simulink library "Prop_demo"  (R2025b)
settings: Solver=VariableStepAuto  StartTime=0.0  StopTime=10.0  RelTol=1e-3
undefined symbols (not defined in the file): cfd2d_ja, cfd2d_jl, cfd2d_kQ, cfd2d_kT, cfd2d_P1_CEF_X, cfd2d_P1_CEF_Y, cfd2d_P1_CEF_Z, cfd2d_P1_CEM_X, cfd2d_P1_CEM_Y, cfd2d_P1_CEM_Z, cfd3d_ja, cfd3d_jl, cfd3d_P2_CEF_X, cfd3d_P2_CEF_Y, cfd3d_P2_CEF_Z, cfd3d_P2_CEM_X, cfd3d_P2_CEM_Y, cfd3d_P2_CEM_Z, cfd3d_pitch, CoefBus, DF3000_V2_Prop, magnitude, Prop1, Prop2
libraries: simulink_extras x7, matrix_library x3, sharedtransform x3, simulink x2, DF3000_V2_Common x1
(part 1 of 2)
settings Model: Creator=someone  LastModifiedBy=someone

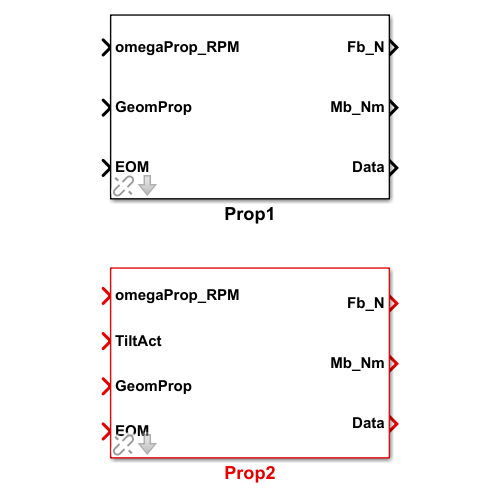
[thumbnail: Simulink's stored preview of the top-level diagram]
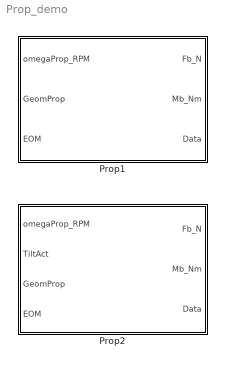
== system Prop_demo ==
  Prop1 : Subsystem  AncestorBlock=DF3000_V2_Prop/Prop1  mask{propAbs=1}
      mask prompts: propAbs "Prop Index"
      mask DialogControl ParameterGroupVar Prompt: 参数
  Prop2 : Subsystem  AncestorBlock=DF3000_V2_Prop/Prop2  mask{propAbs=2, ArmDirSelected=on}
      mask prompts: propAbs "Prop Index"; ArmDirSelected "Positive Installed (Front Prop)"
      mask DialogControl ParameterGroupVar Prompt: 参数

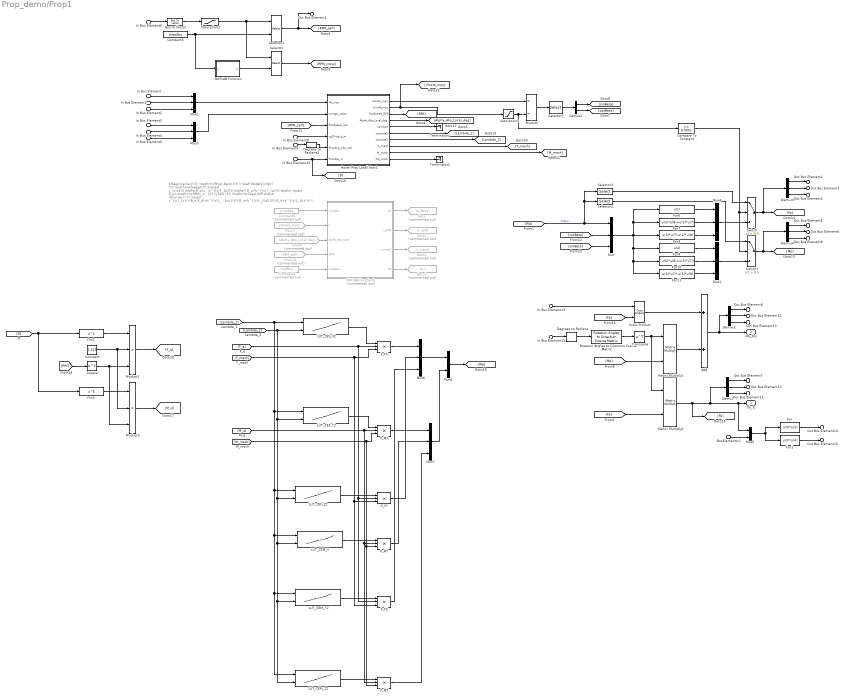
== system Prop_demo/Prop1 ==
  note: $\begin{array}{l} \mathrm{Prop\ Aero\ Fit\ /\ Coef\ Model}\\[3pt] (1)\ \mathrm{Sweep\ fit:}\quad y_{c,p}(V,\alpha,R_p)=a^{(c)}_{p}(V,\alpha)\,R_p+b^{(c)}_{p}(V,\alpha),\quad R_p=\mathrm{RPM}_p^{2}.\\[5pt] (2)\ \mathrm{Coax\ diff\ plane\ (one\ pair):}\\ \quad y^{u}_{c}(V,R_u,R_d)=k^{(c)}_{uu}(V)\,R_u+k^{(c)}_{ud}(V)\,R_d+b^{(c)}_{u}(V),\\ \quad y^{d}_{c}(V,R_u,R_d)=k^{(c)}_{du}(V)\,R_u+k^{(c)}_{dd}(V)\,R_d+b^{(c)}_{d}(V).\\[5pt] (3)\ \mathrm{Ratio\ (split\ of\ slope):}\quad s^{(c)}_{u}=k^{(c)}_{uu}+k^{(c)}_{ud},\quad s^{(c)}_{d}=k^{(c)}_{dd}+k^{(c)}_{du},\\ \quad r^{(c)}_{uu}=\frac{k^{(c)}_{uu}}{s^{(c)}_{u}},\quad r^{(c)}_{ud}=\frac{k^{(c)}_{ud}}{s^{(c)}_{u}},\quad r^{(c)}_{dd}=\frac{k^{(c)}_{dd}}{s^{(c)}_{d}},\quad r^{(c)}_{du}=\frac{k^{(c)}_{du}}{s^{(c)}_{d}}.\\[5pt] (4)\ \mathrm{Coax\ weight:}\quad s=(\cos(\alpha))^{p},\quad p=\mathrm{coaxAlphaPow}.\\ \quad \mathrm{upper:}\quad a^{(c)}_{\mathrm{self}}=s\,r^{(c)}_{uu}\,a^{(c)}_{p},\quad a^{(c)}_{\mathrm{cross}}=s\,r^{(c)}_{ud}\,a^{(c)}_{p},\\ \quad \mathrm{lower:}\quad a^{(c)}_{\mathrm{self}}=s\,r^{(c)}_{dd}\,a^{(c)}_{p},\quad a^{(c)}_{\mathrm{cross}}=s\,r^{(c)}_{du}\,a^{(c)}_{p}.\\[5pt] (5)\ \mathrm{Final\ prediction:}\quad \hat y_{c,p}=a^{(c)}_{\mathrm{self}}\,R_p+a^{(c)}_{\mathrm{cross}}\,R_{m(p)}+b^{(c)}_{p}(V,\alpha). \end{array}$
  In Bus Element6 : Inport  PortName=omegaProp_RPM
      settings: AttributesFormatString=%<OutDataTypeStr>\nDimensions: %<PortDimensions>
  In Bus Element12 : Inport  Port=2  PortName=GeomProp  Element=cg2Prop_b_m
      settings: AttributesFormatString=%<OutDataTypeStr>\nDimensions: %<PortDimensions>
  In Bus Element8 : Inport  Port=2  PortName=GeomProp  Element=cg2Prop_b_m
      settings: AttributesFormatString=%<OutDataTypeStr>\nDimensions: %<PortDimensions>
  In Bus Element13 : Inport  Port=2  PortName=GeomProp  Element=PropAng_b2p_deg
      settings: AttributesFormatString=%<OutDataTypeStr>\nDimensions: %<PortDimensions>
  In Bus Element9 : Inport  Port=2  PortName=GeomProp  Element=PropAng_b2p_deg
      settings: AttributesFormatString=%<OutDataTypeStr>\nDimensions: %<PortDimensions>
  In Bus Element10 : Inport  Port=2  PortName=GeomProp  Element=PropDia_m
      settings: AttributesFormatString=%<OutDataTypeStr>\nDimensions: %<PortDimensions>
  BusElementIn1 : Inport  Port=2  PortName=GeomProp  Element=root2Prop_b_m
  In Bus Element : Inport  Port=3  PortName=EOM  Element=VB_mps.Ub_mps
      settings: AttributesFormatString=%<OutDataTypeStr>\nDimensions: %<PortDimensions>
  In Bus Element1 : Inport  Port=3  PortName=EOM  Element=VB_mps.Vb_mps
      settings: AttributesFormatString=%<OutDataTypeStr>\nDimensions: %<PortDimensions>
  In Bus Element2 : Inport  Port=3  PortName=EOM  Element=VB_mps.Wb_mps
      settings: AttributesFormatString=%<OutDataTypeStr>\nDimensions: %<PortDimensions>
  In Bus Element3 : Inport  Port=3  PortName=EOM  Element=Rates_radps.P_radps
      settings: AttributesFormatString=%<OutDataTypeStr>\nDimensions: %<PortDimensions>
  In Bus Element4 : Inport  Port=3  PortName=EOM  Element=Rates_radps.Q_radps
      settings: AttributesFormatString=%<OutDataTypeStr>\nDimensions: %<PortDimensions>
  In Bus Element5 : Inport  Port=3  PortName=EOM  Element=Rates_radps.R_radps
      settings: AttributesFormatString=%<OutDataTypeStr>\nDimensions: %<PortDimensions>
  Add : Sum
  Bus to Vector : BusToVector
  Compare To Constant : simulink/Logic and Bit Operations/Compare To Constant  relop=<=  const=0.0001  OutDataTypeStr=boolean
  Constant : Constant  Value=1.225
  Constant3 : Constant  Value=propAbs
  Constant4 : Constant  Commented=on  Value=CoefBus  OutDataTypeStr=Bus: CoefBusObj
  Constant5 : Constant  Commented=on  Value=propAbs
  Cross Product : matrix_library/Cross Product
  Degrees to Radians : simulink_extras/Transformations/Degrees to Radians
  Degrees to Radians1 : simulink_extras/Transformations/Degrees to Radians
  Demux{,2..4} (4 alike) : Demux  Outputs=3
  Demux1 : Demux  Outputs=2
  Fcn : Fcn  Expr=u(3)*u(5)
  Fcn1 : Fcn  Expr=u(3)*u(4)
  Fcn10 : Fcn  Expr=u(6)*u(8)+u(5)*u(7)
  Fcn11 : Fcn  Expr=u(6)*u(7)-u(5)*u(8)
  Fcn2 : Fcn  Expr=u^4
  Fcn3 : Fcn  Expr=u^5
  Fcn6 : Fcn  Expr=u(1)
  Fcn7 : Fcn  Expr=u(3)*u(8)+u(2)*u(7)
  Fcn8 : Fcn  Expr=u(3)*u(7)-u(2)*u(8)
  Fcn9 : Fcn  Expr=u(4)
  From14 : From  Commented=on  GotoTag=RPM_self
  From6 : From  Commented=on  GotoTag=Alpha_Abs_Local_deg
  From7 : From  Commented=on  GotoTag=Vmold_mps
  Goto : Goto  Commented=on  GotoTag=a_base
  Goto1 : Goto  Commented=on  GotoTag=r_self
  Goto2 : Goto  Commented=on  GotoTag=r_cross
  Goto3 : Goto  Commented=on  GotoTag=b
  Hover Prop Local Vars1 : Subsystem  AncestorBlock=DF3000_V2_Common/Hover Prop Local Vars1
  LUT_CEF_X2 : Lookup_n-D  BreakpointsForDimension1=cfd2d_ja  BreakpointsForDimension2=cfd2d_jl  BreakpointsForDimension3=[5, 7]  Table=cfd2d_P1_CEF_X  ExtrapMethod=Clip  UseLastTableValue=on  InternalRulePriority=Speed  RndMeth=Simplest
      settings: InputPortMap=u0,u1
  LUT_CEF_Y2 : Lookup_n-D  BreakpointsForDimension1=cfd2d_ja  BreakpointsForDimension2=cfd2d_jl  BreakpointsForDimension3=[5, 7]  Table=cfd2d_P1_CEM_X  ExtrapMethod=Clip  UseLastTableValue=on  InternalRulePriority=Speed  RndMeth=Simplest
      settings: InputPortMap=u0,u1
  LUT_CEF_Z2 : Lookup_n-D  BreakpointsForDimension1=cfd2d_ja  BreakpointsForDimension2=cfd2d_jl  BreakpointsForDimension3=[5, 7]  Table=cfd2d_P1_CEF_Y  ExtrapMethod=Clip  UseLastTableValue=on  InternalRulePriority=Speed  RndMeth=Simplest
      settings: InputPortMap=u0,u1
  LUT_CEM_X : Lookup_n-D  BreakpointsForDimension1=cfd2d_ja  BreakpointsForDimension2=cfd2d_jl  BreakpointsForDimension3=[5, 7]  Table=cfd2d_P1_CEM_Y  ExtrapMethod=Clip  UseLastTableValue=on  InternalRulePriority=Speed  RndMeth=Simplest
      settings: InputPortMap=u0,u1
  LUT_CEM_Y2 : Lookup_n-D  BreakpointsForDimension1=cfd2d_ja  BreakpointsForDimension2=cfd2d_jl  BreakpointsForDimension3=[5, 7]  Table=cfd2d_P1_CEF_Z  ExtrapMethod=Clip  UseLastTableValue=on  InternalRulePriority=Speed  RndMeth=Simplest
      settings: InputPortMap=u0,u1
  LUT_CEM_Z2 : Lookup_n-D  BreakpointsForDimension1=cfd2d_ja  BreakpointsForDimension2=cfd2d_jl  BreakpointsForDimension3=[5, 7]  Table=cfd2d_P1_CEM_Z  ExtrapMethod=Clip  UseLastTableValue=on  InternalRulePriority=Speed  RndMeth=Simplest
      settings: InputPortMap=u0,u1
  MATLAB Function : MATLAB Function  TreatAsAtomicUnit=on
  MATLAB Function2 : MATLAB Function  Commented=on  TreatAsAtomicUnit=on
  Matrix Multiply1 : Product  Multiplication=Matrix(*)
  Matrix Multiply2 : Product  Multiplication=Matrix(*)
  Mux{,1..4,6..7} (7 alike) : Mux  Inputs=3
  Mux5 : Mux  Inputs=2
  Mux8 : Mux  Inputs=2
  P_FX : Product  Inputs=***
  P_FY : Product  Inputs=***
  P_FZ : Product  Inputs=***
  P_MX : Product  Inputs=***
  P_MY : Product  Inputs=***
  P_MZ : Product  Inputs=***
  Product : Product  Inputs=*/
  Product1 : Product  Inputs=3
  Product3 : Product  Inputs=3
  Rotation Angles to Direction Cosine Matrix : sharedtransform/Rotation Angles to Direction Cosine Matrix  rotationOrder=XYZ  aMode=aMode
  Saturation1 : Saturate  UpperLimit=inf  LowerLimit=0.0001
  Saturation2 : Saturate  UpperLimit=1500  LowerLimit=0
      settings: AttributesFormatString=min: %<LowerLimit>\nmax: %<UpperLimit>
  Selector : Selector  InputPortWidth=8  IndexOptions=Index vector (port)  Indices=[1 3]  OutputSizes=1
  Selector1 : Selector  InputPortWidth=8  IndexOptions=Index vector (port)  Indices=[1 3]  OutputSizes=1
  Selector2 : Selector  InputPortWidth=3  IndexOptions=Index vector (dialog)  Indices=[2 3]  OutputSizes=1
  Selector3 : Selector  InputPortWidth=6  IndexOptions=Index vector (dialog)  Indices=[1 2 3]  OutputSizes=1
  Selector4 : Selector  InputPortWidth=6  IndexOptions=Index vector (dialog)  Indices=[4 5 6]  OutputSizes=1
  Square : Math  Operator=square
  Switch : Switch  Criteria=u2 > Threshold  Threshold=0.5  SaturateOnIntegerOverflow=off  InputSameDT=off
  Switch1 : Switch  Criteria=u2 > Threshold  Threshold=0.5  SaturateOnIntegerOverflow=off  InputSameDT=off
  Terminator1 : Terminator
  Terminator2 : Terminator
  Transpose : Math  Operator=transpose
  Fb_N : Outport  PortDimensions=3
  Mb_Nm : Outport  Port=2  PortDimensions=3
  Out Bus Element7 : Outport  Port=3  PortName=Data  Element=Fx_Prop
  Out Bus Element10 : Outport  Port=3  PortName=Data  Element=Fy_Prop
  Out Bus Element11 : Outport  Port=3  PortName=Data  Element=Fz_Prop
  Out Bus Element8 : Outport  Port=3  PortName=Data  Element=Mx_Prop
  Out Bus Element12 : Outport  Port=3  PortName=Data  Element=My_Prop
  Out Bus Element13 : Outport  Port=3  PortName=Data  Element=Mz_Prop
  Out Bus Element1 : Outport  Port=3  PortName=Data  Element=RPM
  Out Bus Element2 : Outport  Port=3  PortName=Data  Element=Fx_Local
  Out Bus Element3 : Outport  Port=3  PortName=Data  Element=Fy_Local
  Out Bus Element4 : Outport  Port=3  PortName=Data  Element=Fz_Local
  Out Bus Element5 : Outport  Port=3  PortName=Data  Element=Mx_Local
  Out Bus Element6 : Outport  Port=3  PortName=Data  Element=My_Local
  Out Bus Element9 : Outport  Port=3  PortName=Data  Element=Mz_Local
  Out Bus Element14 : Outport  Port=3  PortName=Data  Element=BMbx_Prop
  Out Bus Element15 : Outport  Port=3  PortName=Data  Element=BMby_Prop
  wires:
  Fcn1/1 -> Out Bus Element15/1
  Fcn/1 -> Out Bus Element14/1
  Mux5/1 -> Fcn/1, Fcn1/1
  BusElementIn1/1 -> Mux5/2
  From14/1 -> MATLAB Function2/4(RPM)
  Demux4/2 -> Out Bus Element6/1
  Demux4/1 -> Out Bus Element5/1
  Demux4/3 -> Out Bus Element9/1
  Demux3/3 -> Out Bus Element4/1
  Demux3/1 -> Out Bus Element2/1
  Demux3/2 -> Out Bus Element3/1
  Selector3/1 -> Switch/1
  Switch/1 -> [Fp], Demux3/1
  Selector4/1 -> Switch1/1
  Mux4/1 -> Switch/3
  Saturation1/1 -> Product/2, Compare To Constant/1
  Compare To Constant/1 -> Switch/2, Switch1/2
  Mux1/1 -> Switch1/3
  Switch1/1 -> [Mp], Demux4/1
  Demux1/1 -> [sinBeta]
  Demux1/2 -> [cosBeta]
  Selector/1 -> [RPM_cross]
  MATLAB Function/1(y) -> Selector/2
  Constant3/1 -> Selector1/2, MATLAB Function/1(u)
  In Bus Element6/1 -> Bus to Vector/1
  Bus to Vector/1 -> Saturation2/1
  Saturation2/1 -> Selector/1, Selector1/1
  MATLAB Function2/1(a6) -> Goto/1
  Rotation Angles to Direction Cosine Matrix/1 -> Transpose/1
  In Bus Element12/1 -> Cross Product/1
  Cross Product/1 -> Add/1
  In Bus Element13/1 -> Degrees to Radians/1
  Degrees to Radians/1 -> Rotation Angles to Direction Cosine Matrix/1
  Matrix Multiply1/1 -> Add/2
  [Mp] -> Matrix Multiply1/2
  Transpose/1 -> Matrix Multiply2/1, Matrix Multiply1/1
  Selector1/1 -> [RPM_self], Out Bus Element1/1
  In Bus Element8/1 -> Hover Prop Local Vars1/4(cg2Prop_b_m)
  In Bus Element9/1 -> Degrees to Radians1/1
  In Bus Element/1 -> Mux2/1
  In Bus Element5/1 -> Mux3/3
  In Bus Element4/1 -> Mux3/2
  In Bus Element3/1 -> Mux3/1
  In Bus Element2/1 -> Mux2/3
  In Bus Element10/1 -> [D], Hover Prop Local Vars1/6(PropDia_m)
  Mux3/1 -> Hover Prop Local Vars1/2(omega_radps)
  Mux2/1 -> Hover Prop Local Vars1/1(Vb_mps)
  In Bus Element1/1 -> Mux2/2
  [RPM_self] -> Hover Prop Local Vars1/3(RotSpeed_rpm)
  Hover Prop Local Vars1/1(VLocal_mps) -> Product/1
  Hover Prop Local Vars1/2(Vmold_mps) -> [Vmold_mps], Saturation1/1
  Product/1 -> Selector2/1
  Selector2/1 -> Demux1/1
  Hover Prop Local Vars1/3(RotSpeed_RPS) -> [RPS]
  Hover Prop Local Vars1/5(Lambda) -> Terminator1/1
  Constant4/1 -> MATLAB Function2/5(CoefBus)
  Constant5/1 -> MATLAB Function2/1(propAbs)
  MATLAB Function2/4(b6) -> Goto3/1
  MATLAB Function2/3(r_cross6) -> Goto2/1
  MATLAB Function2/2(r_self6) -> Goto1/1
  Hover Prop Local Vars1/4(Alpha_Abs_Local_deg) -> [Alpha_Abs_Local_deg]
  From6/1 -> MATLAB Function2/3(Alpha_abs_local)
  From7/1 -> MATLAB Function2/2(V)
  [cosBeta] -> Mux/2
  [sinBeta] -> Mux/3
  Mux/1 -> Fcn7/1, Fcn6/1, Fcn10/1, Fcn11/1, Fcn9/1, Fcn8/1
  Fcn9/1 -> Mux1/1
  Fcn10/1 -> Mux1/2
  Fcn11/1 -> Mux1/3
  Fcn6/1 -> Mux4/1
  Fcn7/1 -> Mux4/2
  Fcn8/1 -> Mux4/3
  [Fp] -> Matrix Multiply2/2
  Matrix Multiply2/1 -> Demux/1, Fb_N/1, Mux5/1, [Fb]
  [Fb] -> Cross Product/2
  [Wp] -> Mux/1, Selector3/1, Selector4/1  "FMpw"
  Demux/1 -> Out Bus Element7/1
  Demux/2 -> Out Bus Element10/1
  Demux/3 -> Out Bus Element11/1
  Demux2/3 -> Out Bus Element13/1
  Demux2/2 -> Out Bus Element12/1
  Demux2/1 -> Out Bus Element8/1
  Add/1 -> Mb_Nm/1, Demux2/1
  Degrees to Radians1/1 -> Hover Prop Local Vars1/5(PropAng_b2p_rad)
  [RPS] -> Square/1
  Square/1 -> Product3/3, Product1/3
  Product3/1 -> [M_q]
  Constant/1 -> Product3/2, Product1/2
  Product1/1 -> [F_q]
  Fcn2/1 -> Product1/1
  Fcn3/1 -> Product3/1
  LUT_CEM_Z2/1 -> P_MZ/1
  LUT_CEF_Z2/1 -> P_FY/1
  [M_q] -> P_MZ/2, P_MY/2, P_MX/2
  [M_mach] -> P_MZ/3, P_MY/3, P_MX/3
  LUT_CEF_X2/1 -> P_FX/1
  LUT_CEM_Y2/1 -> P_FZ/1
  [Lambda_1] -> LUT_CEM_Z2/1, LUT_CEM_Y2/1, LUT_CEM_X/1, LUT_CEF_Z2/1, LUT_CEF_Y2/1, LUT_CEF_X2/1
  P_FX/1 -> Mux6/1
  [Lambda_2] -> LUT_CEM_Z2/2, LUT_CEM_Y2/2, LUT_CEM_X/2, LUT_CEF_Z2/2, LUT_CEF_Y2/2, LUT_CEF_X2/2
  LUT_CEM_X/1 -> P_MY/1
  P_MX/1 -> Mux7/1
  LUT_CEF_Y2/1 -> P_MX/1
  [F_mach] -> P_FZ/3, P_FY/3, P_FX/3
  [F_q] -> P_FZ/2, P_FY/2, P_FX/2
  Hover Prop Local Vars1/6(Lambda1) -> [Lambda_1]
  Hover Prop Local Vars1/7(Lambda2) -> [Lambda_2]
  Hover Prop Local Vars1/8(F_mach) -> [F_mach]
  Hover Prop Local Vars1/9(M_mach) -> [M_mach]
  Hover Prop Local Vars1/10(Tip_mach) -> Terminator2/1
  P_FY/1 -> Mux6/2
  P_FZ/1 -> Mux6/3
  P_MY/1 -> Mux7/2
  P_MZ/1 -> Mux7/3
  Mux6/1 -> Mux8/1
  Mux7/1 -> Mux8/2
  Mux8/1 -> [Wp]
  [D] -> Fcn3/1, Fcn2/1

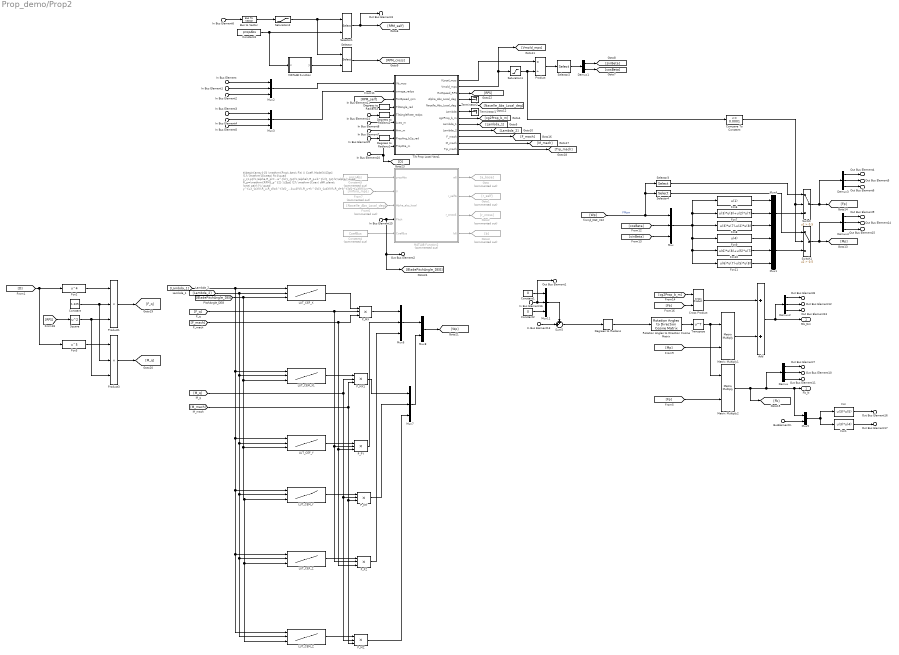
== system Prop_demo/Prop2 ==
  note: $\begin{array}{l} \mathrm{Prop\ Aero\ Fit\ /\ Coef\ Model}\\[3pt] (1)\ \mathrm{Sweep\ fit:}\quad y_{c,p}(V,\alpha,R_p)=a^{(c)}_{p}(V,\alpha)\,R_p+b^{(c)}_{p}(V,\alpha),\quad R_p=\mathrm{RPM}_p^{2}.\\[5pt] (2)\ \mathrm{Coax\ diff\ plane\ (one\ pair):}\\ \quad y^{u}_{c}(V,R_u,R_d)=k^{(c)}_{uu}(V)\,R_u+k^{(c)}_{ud}(V)\,R_d+b^{(c)}_{u}(V),\\ \quad y^{d}_{c}(V,R_u,R_d)=k^{(c)}_{du}(V)\,R_u+k^{(c)}_{dd}(V)\,R_d+b^{(c)}_{d}(V).\\[5pt] (3)\ \mathrm{Ratio\ (split\ of\ slope):}\quad s^{(c)}_{u}=k^{(c)}_{uu}+k^{(c)}_{ud},\quad s^{(c)}_{d}=k^{(c)}_{dd}+k^{(c)}_{du},\\ \quad r^{(c)}_{uu}=\frac{k^{(c)}_{uu}}{s^{(c)}_{u}},\quad r^{(c)}_{ud}=\frac{k^{(c)}_{ud}}{s^{(c)}_{u}},\quad r^{(c)}_{dd}=\frac{k^{(c)}_{dd}}{s^{(c)}_{d}},\quad r^{(c)}_{du}=\frac{k^{(c)}_{du}}{s^{(c)}_{d}}.\\[5pt] (4)\ \mathrm{Coax\ weight:}\quad s=(\cos(\alpha))^{p},\quad p=\mathrm{coaxAlphaPow}.\\ \quad \mathrm{upper:}\quad a^{(c)}_{\mathrm{self}}=s\,r^{(c)}_{uu}\,a^{(c)}_{p},\quad a^{(c)}_{\mathrm{cross}}=s\,r^{(c)}_{ud}\,a^{(c)}_{p},\\ \quad \mathrm{lower:}\quad a^{(c)}_{\mathrm{self}}=s\,r^{(c)}_{dd}\,a^{(c)}_{p},\quad a^{(c)}_{\mathrm{cross}}=s\,r^{(c)}_{du}\,a^{(c)}_{p}.\\[5pt] (5)\ \mathrm{Final\ prediction:}\quad \hat y_{c,p}=a^{(c)}_{\mathrm{self}}\,R_p+a^{(c)}_{\mathrm{cross}}\,R_{m(p)}+b^{(c)}_{p}(V,\alpha). \end{array}$
  In Bus Element6 : Inport  PortName=omegaProp_RPM
      settings: AttributesFormatString=%<OutDataTypeStr>\nDimensions: %<PortDimensions>
  In Bus Element14 : Inport  Port=2  PortName=TiltAct  Element=TiltAngleRate_dps
  In Bus Element15 : Inport  Port=2  PortName=TiltAct  Element=BladePitchAngle_DEG
  In Bus Element11 : Inport  Port=2  PortName=TiltAct  Element=TiltAngle_DEG
  In Bus Element16 : Inport  Port=2  PortName=TiltAct  Element=TiltAngle_DEG
  In Bus Element13 : Inport  Port=3  PortName=GeomProp  Element=PropAng_b2p_deg
      settings: AttributesFormatString=%<OutDataTypeStr>\nDimensions: %<PortDimensions>
  In Bus Element9 : Inport  Port=3  PortName=GeomProp  Element=PropAng_b2p_deg
      settings: AttributesFormatString=%<OutDataTypeStr>\nDimensions: %<PortDimensions>
  In Bus Element10 : Inport  Port=3  PortName=GeomProp  Element=PropDia_m
      settings: AttributesFormatString=%<OutDataTypeStr>\nDimensions: %<PortDimensions>
  In Bus Element8 : Inport  Port=3  PortName=GeomProp  Element=cg2PropHinge_b_m
      settings: AttributesFormatString=%<OutDataTypeStr>\nDimensions: %<PortDimensions>
  BusElementIn : Inport  Port=3  PortName=GeomProp  Element=cg2PropHinge_b_m
  In Bus Element7 : Inport  Port=3  PortName=GeomProp  Element=TiltArm_m
      settings: AttributesFormatString=%<OutDataTypeStr>\nDimensions: %<PortDimensions>
  In Bus Element : Inport  Port=4  PortName=EOM  Element=VB_mps.Ub_mps
      settings: AttributesFormatString=%<OutDataTypeStr>\nDimensions: %<PortDimensions>
  In Bus Element1 : Inport  Port=4  PortName=EOM  Element=VB_mps.Vb_mps
      settings: AttributesFormatString=%<OutDataTypeStr>\nDimensions: %<PortDimensions>
  In Bus Element2 : Inport  Port=4  PortName=EOM  Element=VB_mps.Wb_mps
      settings: AttributesFormatString=%<OutDataTypeStr>\nDimensions: %<PortDimensions>
  In Bus Element3 : Inport  Port=4  PortName=EOM  Element=Rates_radps.P_radps
      settings: AttributesFormatString=%<OutDataTypeStr>\nDimensions: %<PortDimensions>
  In Bus Element4 : Inport  Port=4  PortName=EOM  Element=Rates_radps.Q_radps
      settings: AttributesFormatString=%<OutDataTypeStr>\nDimensions: %<PortDimensions>
  In Bus Element5 : Inport  Port=4  PortName=EOM  Element=Rates_radps.R_radps
      settings: AttributesFormatString=%<OutDataTypeStr>\nDimensions: %<PortDimensions>
  Add : Sum
  Bus to Vector : BusToVector
  Compare To Constant : simulink/Logic and Bit Operations/Compare To Constant  relop=<=  const=0.0001  OutDataTypeStr=boolean
  Constant : Constant  Value=1.225
  Constant1 : Constant  Value=0
  Constant2 : Constant  Value=0
  Constant3 : Constant  Value=propAbs
  Constant4 : Constant  Commented=on  Value=CoefBus  OutDataTypeStr=Bus: CoefBusObj
  Constant5 : Constant  Commented=on  Value=propAbs
  Cross Product : matrix_library/Cross Product
  Degrees to Radians{,1..3} (4 alike) : simulink_extras/Transformations/Degrees to Radians
  Demux{,2..4} (4 alike) : Demux  Outputs=3
  Demux1 : Demux  Outputs=2
  Fcn : Fcn  Expr=u(3)*u(5)
  Fcn1 : Fcn  Expr=u(3)*u(4)
  Fcn10 : Fcn  Expr=u(6)*u(8)+u(5)*u(7)
  Fcn11 : Fcn  Expr=u(6)*u(7)-u(5)*u(8)
  Fcn2 : Fcn  Expr=u^4
  Fcn3 : Fcn  Expr=u^5
  Fcn6 : Fcn  Expr=u(1)
  Fcn7 : Fcn  Expr=u(3)*u(8)+u(2)*u(7)
  Fcn8 : Fcn  Expr=u(3)*u(7)-u(2)*u(8)
  Fcn9 : Fcn  Expr=u(4)
  From6 : From  Commented=on  GotoTag=Nacelle_Abs_Local_deg
  From7 : From  Commented=on  GotoTag=Vmold_mps
  Goto : Goto  Commented=on  GotoTag=a_base
  Goto1 : Goto  Commented=on  GotoTag=r_self
  Goto2 : Goto  Commented=on  GotoTag=r_cross
  Goto3 : Goto  Commented=on  GotoTag=b
  LUT_CEF_X : Lookup_n-D  NumberOfTableDimensions=3  BreakpointsForDimension1=cfd3d_ja  BreakpointsForDimension2=cfd3d_jl  BreakpointsForDimension3=cfd3d_pitch  Table=cfd3d_P2_CEF_X  ExtrapMethod=Clip  UseLastTableValue=on  InternalRulePriority=Speed  RndMeth=Simplest
      settings: InputPortMap=u0,u1,u2
  LUT_CEF_Y : Lookup_n-D  NumberOfTableDimensions=3  BreakpointsForDimension1=cfd3d_ja  BreakpointsForDimension2=cfd3d_jl  BreakpointsForDimension3=cfd3d_pitch  Table=cfd3d_P2_CEF_Y  ExtrapMethod=Clip  UseLastTableValue=on  InternalRulePriority=Speed  RndMeth=Simplest
      settings: InputPortMap=u0,u1,u2
  LUT_CEF_Z : Lookup_n-D  NumberOfTableDimensions=3  BreakpointsForDimension1=cfd3d_ja  BreakpointsForDimension2=cfd3d_jl  BreakpointsForDimension3=cfd3d_pitch  Table=cfd3d_P2_CEF_Z  ExtrapMethod=Clip  UseLastTableValue=on  InternalRulePriority=Speed  RndMeth=Simplest
      settings: InputPortMap=u0,u1,u2
  LUT_CEM_X1 : Lookup_n-D  NumberOfTableDimensions=3  BreakpointsForDimension1=cfd3d_ja  BreakpointsForDimension2=cfd3d_jl  BreakpointsForDimension3=cfd3d_pitch  Table=cfd3d_P2_CEM_X  ExtrapMethod=Clip  UseLastTableValue=on  InternalRulePriority=Speed  RndMeth=Simplest
      settings: InputPortMap=u0,u1,u2
  LUT_CEM_Y : Lookup_n-D  NumberOfTableDimensions=3  BreakpointsForDimension1=cfd3d_ja  BreakpointsForDimension2=cfd3d_jl  BreakpointsForDimension3=cfd3d_pitch  Table=cfd3d_P2_CEM_Y  ExtrapMethod=Clip  UseLastTableValue=on  InternalRulePriority=Speed  RndMeth=Simplest
      settings: InputPortMap=u0,u1,u2
  LUT_CEM_Z : Lookup_n-D  NumberOfTableDimensions=3  BreakpointsForDimension1=cfd3d_ja  BreakpointsForDimension2=cfd3d_jl  BreakpointsForDimension3=cfd3d_pitch  Table=cfd3d_P2_CEM_Z  ExtrapMethod=Clip  UseLastTableValue=on  InternalRulePriority=Speed  RndMeth=Simplest
      settings: InputPortMap=u0,u1,u2
  MATLAB Function : MATLAB Function  TreatAsAtomicUnit=on
  MATLAB Function2 : MATLAB Function  Commented=on  TreatAsAtomicUnit=on
  Matrix Multiply1 : Product  Multiplication=Matrix(*)
  Matrix Multiply2 : Product  Multiplication=Matrix(*)
  Mux{,1..4,6..7,11} (8 alike) : Mux  Inputs=3
  Mux5 : Mux  Inputs=2
  Mux8 : Mux  Inputs=2
  P_FY : Product  Inputs=***
  P_FZ : Product  Inputs=***
  P_MX : Product  Inputs=***
  P_MX1 : Product  Inputs=***
  P_MY : Product  Inputs=***
  P_MZ : Product  Inputs=***
  Product : Product  Inputs=*/
  Product1 : Product  Inputs=3
  Product3 : Product  Inputs=3
  Rotation Angles to Direction Cosine Matrix : sharedtransform/Rotation Angles to Direction Cosine Matrix  rotationOrder=XYZ  aMode=aMode
  Saturation1 : Saturate  UpperLimit=inf  LowerLimit=0.0001
  Saturation2 : Saturate  UpperLimit=1500  LowerLimit=0
      settings: AttributesFormatString=min: %<LowerLimit>\nmax: %<UpperLimit>
  Selector : Selector  InputPortWidth=8  IndexOptions=Index vector (port)  Indices=[1 3]  OutputSizes=1
  Selector1 : Selector  InputPortWidth=8  IndexOptions=Index vector (port)  Indices=[1 3]  OutputSizes=1
  Selector2 : Selector  InputPortWidth=3  IndexOptions=Index vector (dialog)  Indices=[2 3]  OutputSizes=1
  Selector3 : Selector  InputPortWidth=6  IndexOptions=Index vector (dialog)  Indices=[1 2 3]  OutputSizes=1
  Selector4 : Selector  InputPortWidth=6  IndexOptions=Index vector (dialog)  Indices=[4 5 6]  OutputSizes=1
  Square : Math  Operator=square
  Sum5 : Sum  Inputs=++|
  Switch : Switch  Criteria=u2 > Threshold  Threshold=0.5  SaturateOnIntegerOverflow=off  InputSameDT=off
  Switch1 : Switch  Criteria=u2 > Threshold  Threshold=0.5  SaturateOnIntegerOverflow=off  InputSameDT=off
  Terminator1 : Terminator
  Terminator2 : Terminator
  Tilt Prop Local Vars1 : Subsystem  AncestorBlock=DF3000_V2_Common/Tilt Prop Local Vars1
  Transpose : Math  Operator=transpose
  Fb_N : Outport  PortDimensions=3
  Mb_Nm : Outport  Port=2  PortDimensions=3
  Out Bus Element7 : Outport  Port=3  PortName=Data  Element=Fx_Prop
  Out Bus Element10 : Outport  Port=3  PortName=Data  Element=Fy_Prop
  Out Bus Element11 : Outport  Port=3  PortName=Data  Element=Fz_Prop
  Out Bus Element8 : Outport  Port=3  PortName=Data  Element=Mx_Prop
  Out Bus Element12 : Outport  Port=3  PortName=Data  Element=My_Prop
  Out Bus Element13 : Outport  Port=3  PortName=Data  Element=Mz_Prop
  Out Bus Element1 : Outport  Port=3  PortName=Data  Element=TiltAngle_DEG
  Out Bus Element2 : Outport  Port=3  PortName=Data  Element=BladePitchAngle_DEG
  Out Bus Element3 : Outport  Port=3  PortName=Data  Element=RPM
  Out Bus Element4 : Outport  Port=3  PortName=Data  Element=Fx_Local
  Out Bus Element5 : Outport  Port=3  PortName=Data  Element=Fy_Local
  Out Bus Element6 : Outport  Port=3  PortName=Data  Element=Fz_Local
  Out Bus Element9 : Outport  Port=3  PortName=Data  Element=Mx_Local
  Out Bus Element14 : Outport  Port=3  PortName=Data  Element=My_Local
  Out Bus Element15 : Outport  Port=3  PortName=Data  Element=Mz_Local
  Out Bus Element16 : Outport  Port=3  PortName=Data  Element=BMbx_Prop
  Out Bus Element17 : Outport  Port=3  PortName=Data  Element=BMby_Prop
  wires:
  Fcn1/1 -> Out Bus Element17/1
  BusElementIn/1 -> Mux5/2
  Mux5/1 -> Fcn/1, Fcn1/1
  Fcn/1 -> Out Bus Element16/1
  Matrix Multiply2/1 -> [Fb], Fb_N/1, Mux5/1, Demux/1
  Demux4/2 -> Out Bus Element14/1
  Demux4/1 -> Out Bus Element9/1
  Switch1/1 -> [Mp], Demux4/1
  Demux4/3 -> Out Bus Element15/1
  Demux3/2 -> Out Bus Element5/1
  Demux3/1 -> Out Bus Element4/1
  Demux3/3 -> Out Bus Element6/1
  Switch/1 -> [Fp], Demux3/1
  Compare To Constant/1 -> Switch/2, Switch1/2
  Selector4/1 -> Switch1/1
  Selector3/1 -> Switch/1
  Saturation1/1 -> Product/2, Compare To Constant/1
  Tilt Prop Local Vars1/7(cg2Prop_b_m) -> [cg2Prop_b_m]
  Tilt Prop Local Vars1/5(Nacelle_Abs_Local_deg) -> [Nacelle_Abs_Local_deg]
  Tilt Prop Local Vars1/4(Alpha_Abs_Local_deg) -> Terminator2/1
  Demux1/2 -> [cosBeta]
  Demux1/1 -> [sinBeta]
  In Bus Element13/1 -> Sum5/2
  In Bus Element16/1 -> Mux11/2, Out Bus Element1/1
  Constant1/1 -> Mux11/1
  Constant2/1 -> Mux11/3
  Mux11/1 -> Sum5/1
  Add/1 -> Demux2/1, Mb_Nm/1
  Demux2/1 -> Out Bus Element8/1
  Demux2/2 -> Out Bus Element12/1
  Demux2/3 -> Out Bus Element13/1
  Demux/3 -> Out Bus Element11/1
  Demux/2 -> Out Bus Element10/1
  Demux/1 -> Out Bus Element7/1
  [Wp] -> Mux/1, Selector3/1, Selector4/1  "FMpw"
  [Fb] -> Cross Product/2
  [Fp] -> Matrix Multiply2/2
  Mux4/1 -> Switch/3
  Fcn8/1 -> Mux4/3
  Fcn7/1 -> Mux4/2
  Fcn6/1 -> Mux4/1
  Mux1/1 -> Switch1/3
  Fcn11/1 -> Mux1/3
  Fcn10/1 -> Mux1/2
  Fcn9/1 -> Mux1/1
  Mux/1 -> Fcn10/1, Fcn11/1, Fcn9/1, Fcn6/1, Fcn7/1, Fcn8/1
  [sinBeta] -> Mux/3
  [cosBeta] -> Mux/2
  From7/1 -> MATLAB Function2/2(V)
  From6/1 -> MATLAB Function2/3(Alpha_abs_local)
  MATLAB Function2/2(r_self6) -> Goto1/1
  MATLAB Function2/3(r_cross6) -> Goto2/1
  MATLAB Function2/4(b6) -> Goto3/1
  Constant5/1 -> MATLAB Function2/1(propAbs)
  Constant4/1 -> MATLAB Function2/5(CoefBus)
  Tilt Prop Local Vars1/6(Lambda) -> Terminator1/1
  Tilt Prop Local Vars1/3(RotSpeed_RPS) -> [RPS]
  Selector2/1 -> Demux1/1
  Product/1 -> Selector2/1
  Tilt Prop Local Vars1/2(Vmold_mps) -> [Vmold_mps], Saturation1/1
  Tilt Prop Local Vars1/1(VLocal_mps) -> Product/1
  [RPM_self] -> Tilt Prop Local Vars1/3(RotSpeed_rpm)
  In Bus Element1/1 -> Mux2/2
  Mux2/1 -> Tilt Prop Local Vars1/1(Vb_mps)
  Mux3/1 -> Tilt Prop Local Vars1/2(omega_radps)
  In Bus Element10/1 -> [D], Tilt Prop Local Vars1/9(PropDia_m)
  In Bus Element2/1 -> Mux2/3
  In Bus Element3/1 -> Mux3/1
  In Bus Element4/1 -> Mux3/2
  In Bus Element5/1 -> Mux3/3
  In Bus Element/1 -> Mux2/1
  In Bus Element9/1 -> Degrees to Radians1/1
  In Bus Element8/1 -> Tilt Prop Local Vars1/6(Lvec_m)
  Selector1/1 -> [RPM_self], Out Bus Element3/1
  Transpose/1 -> Matrix Multiply1/1, Matrix Multiply2/1
  [Mp] -> Matrix Multiply1/2
  Matrix Multiply1/1 -> Add/2
  Degrees to Radians/1 -> Rotation Angles to Direction Cosine Matrix/1
  Sum5/1 -> Degrees to Radians/1
  Cross Product/1 -> Add/1
  [cg2Prop_b_m] -> Cross Product/1
  Rotation Angles to Direction Cosine Matrix/1 -> Transpose/1
  MATLAB Function2/1(a6) -> Goto/1
  Saturation2/1 -> Selector1/1, Selector/1
  Bus to Vector/1 -> Saturation2/1
  In Bus Element6/1 -> Bus to Vector/1
  Constant3/1 -> MATLAB Function/1(u), Selector1/2
  MATLAB Function/1(y) -> Selector/2
  Selector/1 -> [RPM_cross]
  Degrees to Radians1/1 -> Tilt Prop Local Vars1/8(PropAng_b2p_rad)
  In Bus Element7/1 -> Tilt Prop Local Vars1/7(Arm_m)
  Degrees to Radians3/1 -> Tilt Prop Local Vars1/4(TiltAngle_rad)
  Degrees to Radians2/1 -> Tilt Prop Local Vars1/5(TiltAngleRate_radps)
  In Bus Element14/1 -> Degrees to Radians2/1
  In Bus Element11/1 -> Degrees to Radians3/1
  In Bus Element15/1 -> MATLAB Function2/4(Pitch), [BladePitchAngle_DEG], Out Bus Element2/1
  Tilt Prop Local Vars1/8(Lambda_1) -> [Lambda_1]
  Tilt Prop Local Vars1/9(Lambda_2) -> [Lambda_2]
  Tilt Prop Local Vars1/10(F_mach) -> [F_mach]
  Tilt Prop Local Vars1/11(M_mach) -> [M_mach]
  Tilt Prop Local Vars1/12(Tip_mach) -> [Tip_mach]
  [F_q] -> P_MX/2, P_FZ/2, P_FY/2
  [M_mach] -> P_MX1/3, P_MZ/3, P_MY/3
  LUT_CEF_Y/1 -> P_FY/1
  [F_mach] -> P_MX/3, P_FZ/3, P_FY/3
  LUT_CEM_Z/1 -> P_MZ/1
  LUT_CEM_Y/1 -> P_MY/1
  LUT_CEM_X1/1 -> P_MX1/1
  [M_q] -> P_MZ/2, P_MY/2, P_MX1/2
  [Lambda_2] -> LUT_CEM_Z/2, LUT_CEF_Z/2, LUT_CEM_Y/2, LUT_CEF_Y/2, LUT_CEM_X1/2, LUT_CEF_X/2
  [Lambda_1] -> LUT_CEF_X/1, LUT_CEM_Z/1, LUT_CEF_Z/1, LUT_CEM_Y/1, LUT_CEF_Y/1, LUT_CEM_X1/1
  [BladePitchAngle_DEG] -> LUT_CEM_Z/3, LUT_CEF_Z/3, LUT_CEM_Y/3, LUT_CEF_Y/3, LUT_CEM_X1/3, LUT_CEF_X/3
  LUT_CEF_Z/1 -> P_FZ/1
  LUT_CEF_X/1 -> P_MX/1
  P_MX/1 -> Mux6/1
  P_MY/1 -> Mux7/2
  P_MZ/1 -> Mux7/3
  P_FY/1 -> Mux6/2
  Mux6/1 -> Mux8/1
  Mux7/1 -> Mux8/2
  Mux8/1 -> [Wp]
  P_FZ/1 -> Mux6/3
  P_MX1/1 -> Mux7/1
  Fcn2/1 -> Product1/1
  [D] -> Fcn3/1, Fcn2/1
  Fcn3/1 -> Product3/1
  Product1/1 -> [F_q]
  Product3/1 -> [M_q]
  Square/1 -> Product3/3, Product1/3
  Constant/1 -> Product3/2, Product1/2
  [RPS] -> Square/1

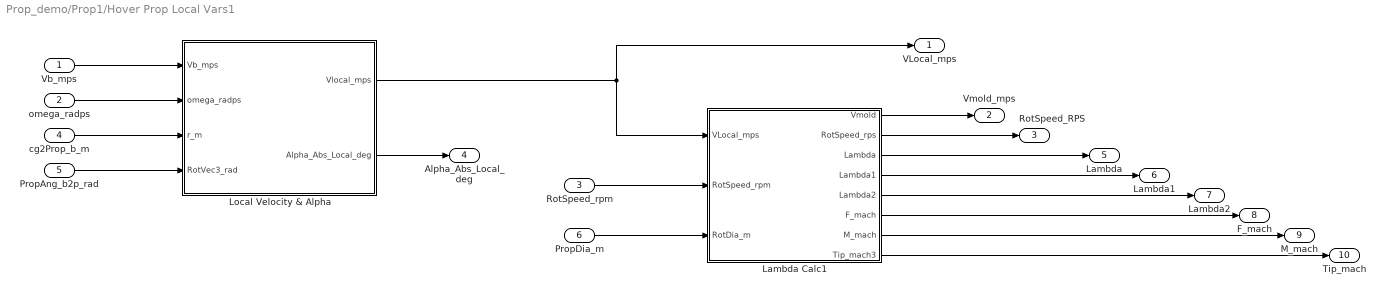
== system Prop_demo/Prop1/Hover Prop Local Vars1 ==
  Vb_mps : Inport
  omega_radps : Inport  Port=2
  RotSpeed_rpm : Inport  Port=3
  cg2Prop_b_m : Inport  Port=4
  PropAng_b2p_rad : Inport  Port=5
  PropDia_m : Inport  Port=6
  Lambda Calc1 : Subsystem  AncestorBlock=DF3000_V2_Common/Lambda Calc1
  Local Velocity & Alpha : Subsystem
  VLocal_mps : Outport
  Vmold_mps : Outport  Port=2
  RotSpeed_RPS : Outport  Port=3
  Alpha_Abs_Local_deg : Outport  Port=4
  Lambda : Outport  Port=5
  Lambda1 : Outport  Port=6
  Lambda2 : Outport  Port=7
  F_mach : Outport  Port=8
  M_mach : Outport  Port=9
  Tip_mach : Outport  Port=10
  wires:
  Lambda Calc1/1(Vmold) -> Vmold_mps/1
  Lambda Calc1/2(RotSpeed_rps) -> RotSpeed_RPS/1
  Lambda Calc1/3(Lambda) -> Lambda/1
  PropDia_m/1 -> Lambda Calc1/3(RotDia_m)
  cg2Prop_b_m/1 -> Local Velocity & Alpha/3(r_m)
  PropAng_b2p_rad/1 -> Local Velocity & Alpha/4(RotVec3_rad)
  Local Velocity & Alpha/2(Alpha_Abs_Local_deg) -> Alpha_Abs_Local_deg/1
  Vb_mps/1 -> Local Velocity & Alpha/1(Vb_mps)
  Local Velocity & Alpha/1(Vlocal_mps) -> VLocal_mps/1, Lambda Calc1/1(VLocal_mps)
  RotSpeed_rpm/1 -> Lambda Calc1/2(RotSpeed_rpm)
  omega_radps/1 -> Local Velocity & Alpha/2(omega_radps)
  Lambda Calc1/4(Lambda1) -> Lambda1/1
  Lambda Calc1/5(Lambda2) -> Lambda2/1
  Lambda Calc1/6(F_mach) -> F_mach/1
  Lambda Calc1/7(M_mach) -> M_mach/1
  Lambda Calc1/8(Tip_mach3) -> Tip_mach/1

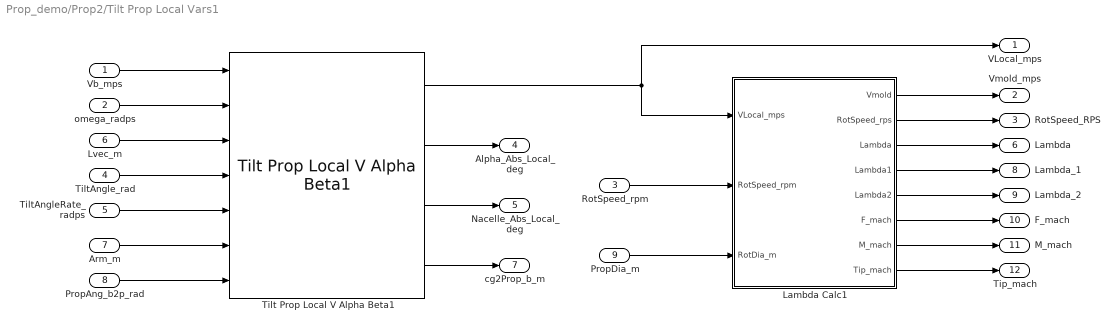
== system Prop_demo/Prop2/Tilt Prop Local Vars1 ==
  Vb_mps : Inport
  omega_radps : Inport  Port=2
  RotSpeed_rpm : Inport  Port=3
  TiltAngle_rad : Inport  Port=4
  TiltAngleRate_radps : Inport  Port=5
  Lvec_m : Inport  Port=6
  Arm_m : Inport  Port=7
  PropAng_b2p_rad : Inport  Port=8
  PropDia_m : Inport  Port=9
  Lambda Calc1 : Subsystem  AncestorBlock=DF3000_V2_Common/Lambda Calc1
  Tilt Prop Local V Alpha Beta1 : DF3000_V2_Common/Tilt Prop Local V Alpha Beta1  SystemSampleTime=-1  VariantActivationTime=update diagram  EmptyChoice=off  PassThrough=off  PassThroughVariantControl=(default)  EmptyChoiceVariantControl=(default)  AllowFlexibleInterface=on  Latency=0  AutoFrameSizeCalculation=off
  VLocal_mps : Outport
  Vmold_mps : Outport  Port=2
  RotSpeed_RPS : Outport  Port=3
  Alpha_Abs_Local_deg : Outport  Port=4
  Nacelle_Abs_Local_deg : Outport  Port=5
  Lambda : Outport  Port=6
  cg2Prop_b_m : Outport  Port=7
  Lambda_1 : Outport  Port=8
  Lambda_2 : Outport  Port=9
  F_mach : Outport  Port=10
  M_mach : Outport  Port=11
  Tip_mach : Outport  Port=12
  wires:
  Lvec_m/1 -> Tilt Prop Local V Alpha Beta1/3
  TiltAngleRate_radps/1 -> Tilt Prop Local V Alpha Beta1/5
  TiltAngle_rad/1 -> Tilt Prop Local V Alpha Beta1/4
  PropAng_b2p_rad/1 -> Tilt Prop Local V Alpha Beta1/7
  Arm_m/1 -> Tilt Prop Local V Alpha Beta1/6
  omega_radps/1 -> Tilt Prop Local V Alpha Beta1/2
  RotSpeed_rpm/1 -> Lambda Calc1/2(RotSpeed_rpm)
  PropDia_m/1 -> Lambda Calc1/3(RotDia_m)
  Tilt Prop Local V Alpha Beta1/1 -> VLocal_mps/1, Lambda Calc1/1(VLocal_mps)
  Vb_mps/1 -> Tilt Prop Local V Alpha Beta1/1
  Tilt Prop Local V Alpha Beta1/2 -> Alpha_Abs_Local_deg/1
  Lambda Calc1/3(Lambda) -> Lambda/1
  Lambda Calc1/2(RotSpeed_rps) -> RotSpeed_RPS/1
  Lambda Calc1/1(Vmold) -> Vmold_mps/1
  Tilt Prop Local V Alpha Beta1/3 -> Nacelle_Abs_Local_deg/1
  Tilt Prop Local V Alpha Beta1/4 -> cg2Prop_b_m/1
  Lambda Calc1/4(Lambda1) -> Lambda_1/1
  Lambda Calc1/5(Lambda2) -> Lambda_2/1
  Lambda Calc1/6(F_mach) -> F_mach/1
  Lambda Calc1/7(M_mach) -> M_mach/1
  Lambda Calc1/8(Tip_mach) -> Tip_mach/1

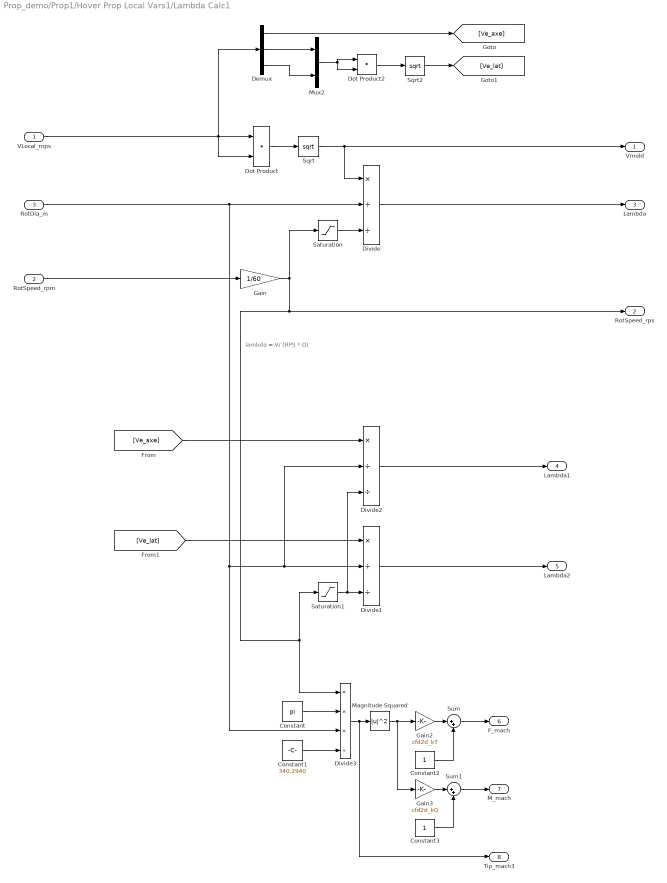
== system Prop_demo/Prop1/Hover Prop Local Vars1/Lambda Calc1 ==
  note: lambda = V/ (RPS * D)
  VLocal_mps : Inport
  RotSpeed_rpm : Inport  Port=2
  RotDia_m : Inport  Port=3
  Constant : Constant  Value=pi
  Constant1 : Constant  Value=340.2940
  Constant2 : Constant
  Constant3 : Constant
  Demux : Demux  Outputs=3
  Divide : Product  Inputs=*//
  Divide1 : Product  Inputs=*//
  Divide2 : Product  Inputs=*//
  Divide3 : Product  Inputs=***/
  Dot Product : DotProduct  OutDataTypeStr=Inherit: Inherit via internal rule
  Dot Product2 : DotProduct  OutDataTypeStr=Inherit: Inherit via internal rule
  Gain : Gain  Gain=1/60
  Gain2 : Gain  Gain=cfd2d_kT
  Gain3 : Gain  Gain=cfd2d_kQ
  Magnitude Squared : Math  Operator=magnitude^2
  Mux2 : Mux  Inputs=2
  Saturation : Saturate  UpperLimit=10000  LowerLimit=0.0001
  Saturation1 : Saturate  UpperLimit=10000  LowerLimit=0.0001
  Sqrt : Sqrt
  Sqrt2 : Sqrt
  Sum : Sum  Inputs=|++
  Sum1 : Sum  Inputs=|++
  Vmold : Outport
  RotSpeed_rps : Outport  Port=2
  Lambda : Outport  Port=3
  Lambda1 : Outport  Port=4
  Lambda2 : Outport  Port=5
  F_mach : Outport  Port=6
  M_mach : Outport  Port=7
  Tip_mach3 : Outport  Port=8
  wires:
  Sqrt/1 -> Divide/1, Vmold/1
  Saturation/1 -> Divide/3
  Dot Product/1 -> Sqrt/1
  VLocal_mps/1 -> Demux/1, Dot Product/1, Dot Product/2
  Divide/1 -> Lambda/1
  RotSpeed_rpm/1 -> Gain/1
  Saturation1/1 -> Divide2/3, Divide1/3
  Gain2/1 -> Sum/1
  Constant/1 -> Divide3/2
  Gain/1 -> Saturation/1, RotSpeed_rps/1, Divide3/1, Saturation1/1
  Constant2/1 -> Sum/2
  [Ve_axe] -> Divide2/1
  Divide3/1 -> Tip_mach3/1, Magnitude Squared/1
  Magnitude Squared/1 -> Gain3/1, Gain2/1
  RotDia_m/1 -> Divide3/3, Divide2/2, Divide1/2, Divide/2
  Constant3/1 -> Sum1/2
  Constant1/1 -> Divide3/4
  Gain3/1 -> Sum1/1
  [Ve_lat] -> Divide1/1
  Dot Product2/1 -> Sqrt2/1
  Demux/2 -> Mux2/1
  Demux/1 -> [Ve_axe]
  Demux/3 -> Mux2/2
  Mux2/1 -> Dot Product2/2, Dot Product2/1
  Sqrt2/1 -> [Ve_lat]
  Divide2/1 -> Lambda1/1
  Divide1/1 -> Lambda2/1
  Sum/1 -> F_mach/1
  Sum1/1 -> M_mach/1

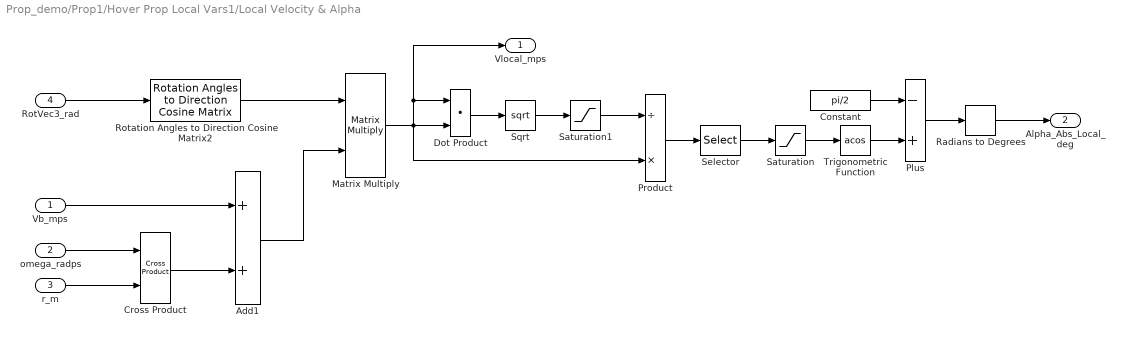
== system Prop_demo/Prop1/Hover Prop Local Vars1/Local Velocity & Alpha ==
  Vb_mps : Inport
  omega_radps : Inport  Port=2
  r_m : Inport  Port=3
  RotVec3_rad : Inport  Port=4
  Add1 : Sum
  Constant : Constant  Value=pi/2
  Cross Product : matrix_library/Cross Product
  Dot Product : DotProduct  OutDataTypeStr=Inherit: Inherit via internal rule
  Matrix Multiply : Product  Multiplication=Matrix(*)
  Plus : Sum  Inputs=-+
  Product : Product  Inputs=/*
  Radians to Degrees : simulink_extras/Transformations/Radians to Degrees
  Rotation Angles to Direction Cosine Matrix2 : sharedtransform/Rotation Angles to Direction Cosine Matrix  rotationOrder=XYZ  aMode=aMode
  Saturation : Saturate  UpperLimit=1  LowerLimit=-1
  Saturation1 : Saturate  UpperLimit=inf  LowerLimit=0.0001
  Selector : Selector  InputPortWidth=3  IndexOptions=Index vector (dialog)  Indices=[1]  OutputSizes=1
  Sqrt : Sqrt
  Trigonometric Function : Trigonometry  Operator=acos
  Vlocal_mps : Outport
  Alpha_Abs_Local_deg : Outport  Port=2
  wires:
  RotVec3_rad/1 -> Rotation Angles to Direction Cosine Matrix2/1
  Rotation Angles to Direction Cosine Matrix2/1 -> Matrix Multiply/1
  Matrix Multiply/1 -> Product/2, Vlocal_mps/1, Dot Product/1, Dot Product/2
  omega_radps/1 -> Cross Product/1
  r_m/1 -> Cross Product/2
  Cross Product/1 -> Add1/2
  Add1/1 -> Matrix Multiply/2
  Vb_mps/1 -> Add1/1
  Dot Product/1 -> Sqrt/1
  Sqrt/1 -> Saturation1/1
  Product/1 -> Selector/1
  Selector/1 -> Saturation/1
  Saturation/1 -> Trigonometric Function/1
  Radians to Degrees/1 -> Alpha_Abs_Local_deg/1
  Trigonometric Function/1 -> Plus/2
  Constant/1 -> Plus/1
  Plus/1 -> Radians to Degrees/1
  Saturation1/1 -> Product/1

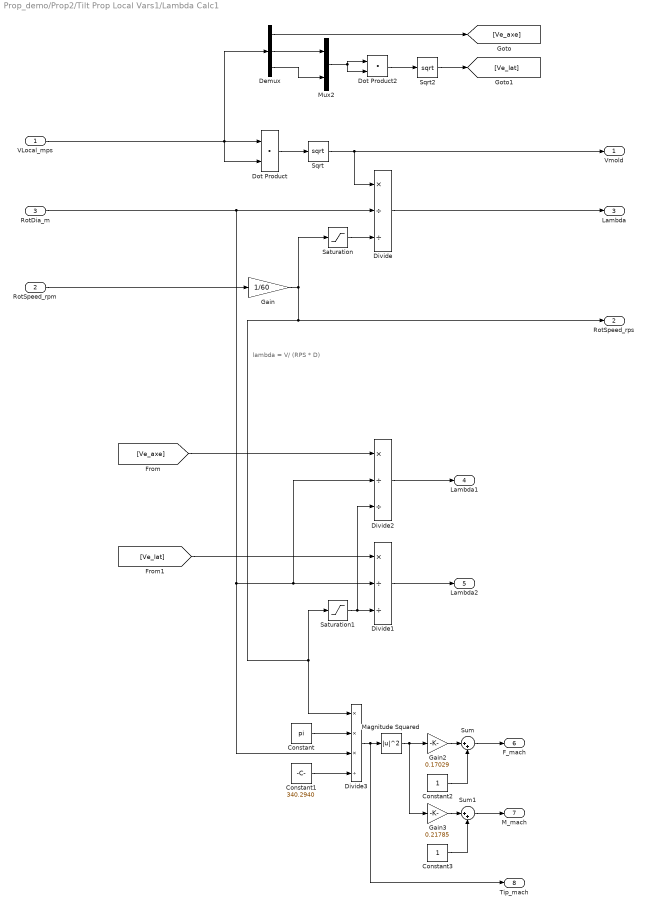
== system Prop_demo/Prop2/Tilt Prop Local Vars1/Lambda Calc1 ==
  note: lambda = V/ (RPS * D)
  VLocal_mps : Inport
  RotSpeed_rpm : Inport  Port=2
  RotDia_m : Inport  Port=3
  Constant : Constant  Value=pi
  Constant1 : Constant  Value=340.2940
  Constant2 : Constant
  Constant3 : Constant
  Demux : Demux  Outputs=3
  Divide : Product  Inputs=*//
  Divide1 : Product  Inputs=*//
  Divide2 : Product  Inputs=*//
  Divide3 : Product  Inputs=***/
  Dot Product : DotProduct  OutDataTypeStr=Inherit: Inherit via internal rule
  Dot Product2 : DotProduct  OutDataTypeStr=Inherit: Inherit via internal rule
  Gain : Gain  Gain=1/60
  Gain2 : Gain  Gain=0.17029
  Gain3 : Gain  Gain=0.21785
  Magnitude Squared : Math  Operator=magnitude^2
  Mux2 : Mux  Inputs=2
  Saturation : Saturate  UpperLimit=10000  LowerLimit=0.0001
  Saturation1 : Saturate  UpperLimit=10000  LowerLimit=0.0001
  Sqrt : Sqrt
  Sqrt2 : Sqrt
  Sum : Sum  Inputs=|++
  Sum1 : Sum  Inputs=|++
  Vmold : Outport
  RotSpeed_rps : Outport  Port=2
  Lambda : Outport  Port=3
  Lambda1 : Outport  Port=4
  Lambda2 : Outport  Port=5
  F_mach : Outport  Port=6
  M_mach : Outport  Port=7
  Tip_mach : Outport  Port=8
  wires:
  Demux/1 -> [Ve_axe]
  Sum/1 -> F_mach/1
  Demux/2 -> Mux2/1
  Divide2/1 -> Lambda1/1
  [Ve_axe] -> Divide2/1
  Constant1/1 -> Divide3/4
  Constant3/1 -> Sum1/2
  Gain3/1 -> Sum1/1
  Demux/3 -> Mux2/2
  Divide1/1 -> Lambda2/1
  Divide3/1 -> Tip_mach/1, Magnitude Squared/1
  [Ve_lat] -> Divide1/1
  Saturation1/1 -> Divide2/3, Divide1/3
  Constant/1 -> Divide3/2
  Gain2/1 -> Sum/1
  Constant2/1 -> Sum/2
  Mux2/1 -> Dot Product2/2, Dot Product2/1
  VLocal_mps/1 -> Demux/1, Dot Product/1, Dot Product/2
  Dot Product2/1 -> Sqrt2/1
  RotDia_m/1 -> Divide3/3, Divide2/2, Divide1/2, Divide/2
  Dot Product/1 -> Sqrt/1
  Magnitude Squared/1 -> Gain3/1, Gain2/1
  RotSpeed_rpm/1 -> Gain/1
  Gain/1 -> Saturation/1, RotSpeed_rps/1, Divide3/1, Saturation1/1
  Saturation/1 -> Divide/3
  Sqrt/1 -> Vmold/1, Divide/1
  Sqrt2/1 -> [Ve_lat]
  Sum1/1 -> M_mach/1
  Divide/1 -> Lambda/1

== matlab function Prop_demo/Prop1/MATLAB Function ==
  data: u input; y output
function y = mate(u)

if u <= 4
    y = u+4;
else
    y = u-4;
end

== matlab function Prop_demo/Prop2/MATLAB Function ==
  data: u input; y output
function y = mate(u)

if u <= 4
    y = u+4;
else
    y = u-4;
end

== matlab function Prop_demo/Prop1/MATLAB Function2 ==
  data: propAbs input; a6 output; r_self6 output; r_cross6 output; V input; Alpha_abs_local input; RPM input; b6 output; CoefBus input
function [a6, r_self6, r_cross6, b6] = CoefQuery_DF3000_Bus( ...
    propAbs, V, Alpha_abs_local, RPM, CoefBus)
%#codegen
% Pitch is tilt-prop pitch for P2/P3/P6/P7 and actual RPM for hover props.
% The hover low-RPM branch returns direct load in b6 and zero a6.

a6       = zeros(6,1);
b6       = zeros(6,1);
r_self6  = ones(6,1);
r_cross6 = zeros(6,1);

p = int32(propAbs);
if p < 1 || p > 8
    return;
end

isTilt = (p==2) || (p==3) || (p==6) || (p==7);

sgnFy = 1.0;
sgnMx = 1.0;
sgnMz = 1.0;
if (p==3) || (p==4) || (p==7) || (p==8)
    sgnFy = -1.0;
    sgnMx = -1.0;
    sgnMz = -1.0;
end

if isTilt
    Nac = Alpha_abs_local;
    baseK = int32(1);
    if (p==6) || (p==7)
        baseK = int32(2);
    end

    bpV = CoefBus.bpV_t;
    bpP = CoefBus.bpPitch_t;
    bpN = CoefBus.bpNac_t;

    aFx = interp3_trilin(bpV,bpP,bpN, CoefBus.aT_FX(:,:,:,baseK), V, RPM, Nac);
    aFy = interp3_trilin(bpV,bpP,bpN, CoefBus.aT_FY(:,:,:,baseK), V, RPM, Nac);
    aFz = interp3_trilin(bpV,bpP,bpN, CoefBus.aT_FZ(:,:,:,baseK), V, RPM, Nac);
    aMx = interp3_trilin(bpV,bpP,bpN, CoefBus.aT_MX(:,:,:,baseK), V, RPM, Nac);
    aMy = interp3_trilin(bpV,bpP,bpN, CoefBus.aT_MY(:,:,:,baseK), V, RPM, Nac);
    aMz = interp3_trilin(bpV,bpP,bpN, CoefBus.aT_MZ(:,:,:,baseK), V, RPM, Nac);

    bFx = interp3_trilin(bpV,bpP,bpN, CoefBus.bT_FX(:,:,:,baseK), V, RPM, Nac);
    bFy = interp3_trilin(bpV,bpP,bpN, CoefBus.bT_FY(:,:,:,baseK), V, RPM, Nac);
    bFz = interp3_trilin(bpV,bpP,bpN, CoefBus.bT_FZ(:,:,:,baseK), V, RPM, Nac);
    bMx = interp3_trilin(bpV,bpP,bpN, CoefBus.bT_MX(:,:,:,baseK), V, RPM, Nac);
    bMy = interp3_trilin(bpV,bpP,bpN, CoefBus.bT_MY(:,:,:,baseK), V, RPM, Nac);
    bMz = interp3_trilin(bpV,bpP,bpN, CoefBus.bT_MZ(:,:,:,baseK), V, RPM, Nac);
else
    Alpha = Alpha_abs_local;
    RPM = max(double(RPM), 0.0);
    baseK = int32(1);
    if (p==5) || (p==8)
        baseK = int32(2);
    end

    bpV = CoefBus.bpV_h;
    bpA = CoefBus.bpA_h;
    rpmJoin = interp1_clamped(bpV, ...
        CoefBus.hoverLowRpmJoinRPM(:,baseK), V);
    useLowRpm = (CoefBus.hoverLowRpmEnable > 0.5) && (RPM < rpmJoin);

    if useLowRpm
        rpm2 = RPM * RPM;
        bpU = CoefBus.bpRPM2_h_low;
        aFx = 0.0; aFy = 0.0; aFz = 0.0;
        aMx = 0.0; aMy = 0.0; aMz = 0.0;
        bFx = interp3_trilin(bpV,bpA,bpU, CoefBus.lowH_FX(:,:,:,baseK), V, Alpha, rpm2);
        bFy = interp3_trilin(bpV,bpA,bpU, CoefBus.lowH_FY(:,:,:,baseK), V, Alpha, rpm2);
        bFz = interp3_trilin(bpV,bpA,bpU, CoefBus.lowH_FZ(:,:,:,baseK), V, Alpha, rpm2);
        bMx = interp3_trilin(bpV,bpA,bpU, CoefBus.lowH_MX(:,:,:,baseK), V, Alpha, rpm2);
        bMy = interp3_trilin(bpV,bpA,bpU, CoefBus.lowH_MY(:,:,:,baseK), V, Alpha, rpm2);
        bMz = interp3_trilin(bpV,bpA,bpU, CoefBus.lowH_MZ(:,:,:,baseK), V, Alpha, rpm2);
    else
        aFx = interp2_bilin(bpV,bpA, CoefBus.aH_FX(:,:,baseK), V, Alpha);
        aFy = interp2_bilin(bpV,bpA, CoefBus.aH_FY(:,:,baseK), V, Alpha);
        aFz = interp2_bilin(bpV,bpA, CoefBus.aH_FZ(:,:,baseK), V, Alpha);
        aMx = interp2_bilin(bpV,bpA, CoefBus.aH_MX(:,:,baseK), V, Alpha);
        aMy = interp2_bilin(bpV,bpA, CoefBus.aH_MY(:,:,baseK), V, Alpha);
        aMz = interp2_bilin(bpV,bpA, CoefBus.aH_MZ(:,:,baseK), V, Alpha);

        bFx = interp2_bilin(bpV,bpA, CoefBus.bH_FX(:,:,baseK), V, Alpha);
        bFy = interp2_bilin(bpV,bpA, CoefBus.bH_FY(:,:,baseK), V, Alpha);
        bFz = interp2_bilin(bpV,bpA, CoefBus.bH_FZ(:,:,baseK), V, Alpha);
        bMx = interp2_bilin(bpV,bpA, CoefBus.bH_MX(:,:,baseK), V, Alpha);
        bMy = interp2_bilin(bpV,bpA, CoefBus.bH_MY(:,:,baseK), V, Alpha);
        bMz = interp2_bilin(bpV,bpA, CoefBus.bH_MZ(:,:,baseK), V, Alpha);
    end
end

a6(1)=aFx;
a6(2)=sgnFy*aFy;
a6(3)=aFz;
a6(4)=sgnMx*aMx;
a6(5)=aMy;
a6(6)=sgnMz*aMz;

b6(1)=bFx;
b6(2)=sgnFy*bFy;
b6(3)=bFz;
b6(4)=sgnMx*bMx;
b6(5)=bMy;
b6(6)=sgnMz*bMz;
end

function z = interp1_clamped(x,F,xq)
x=double(x(:));
F=double(F(:));
xq=double(xq);
n=numel(x);
if n<2
    z=F(1);
    return;
end
if xq<=x(1)
    z=F(1);
    return;
elseif xq>=x(n)
    z=F(n);
    return;
end
i=1;
while i<n && xq>x(i+1)
    i=i+1;
end
if i>=n
    i=n-1;
end
t=0;
if x(i+1)>x(i)
    t=(xq-x(i))/(x(i+1)-x(i));
end
z=(1-t)*F(i)+t*F(i+1);
end

function z = interp2_bilin(x,y,F,xq,yq)
x=double(x(:));
y=double(y(:));
F=double(F);
xq=double(xq);
yq=double(yq);
nV=numel(x);
nA=numel(y);
if nV<2||nA<2
    z=F(1,1);
    return;
end
if xq<=x(1)
    i=1;
elseif xq>=x(nV)
    i=nV-1;
else
    i=1;
    while i<nV && xq>x(i+1)
        i=i+1;
    end
    if i>=nV
        i=nV-1;
    end
end
if yq<=y(1)
    j=1;
elseif yq>=y(nA)
    j=nA-1;
else
    j=1;
    while j<nA && yq>y(j+1)
        j=j+1;
    end
    if j>=nA
        j=nA-1;
    end
end
tx=0;
if x(i+1)>x(i)
    tx=(xq-x(i))/(x(i+1)-x(i));
end
ty=0;
if y(j+1)>y(j)
    ty=(yq-y(j))/(y(j+1)-y(j));
end
F11=F(i,j);
F12=F(i,j+1);
F21=F(i+1,j);
F22=F(i+1,j+1);
z=(1-tx)*((1-ty)*F11+ty*F12)+tx*((1-ty)*F21+ty*F22);
end

function v = interp3_trilin(x,y,z,F,xq,yq,zq)
x=double(x(:));
y=double(y(:));
z=double(z(:));
F=double(F);
xq=double(xq);
yq=double(yq);
zq=double(zq);
nx=numel(x);
ny=numel(y);
nz=numel(z);
if nx<2||ny<2||nz<2
    v=F(1,1,1);
    return;
end
if xq<=x(1)
    i=1;
elseif xq>=x(nx)
    i=nx-1;
else
    i=1;
    while i<nx && xq>x(i+1)
        i=i+1;
    end
    if i>=nx
        i=nx-1;
    end
end
if yq<=y(1)
    j=1;
elseif yq>=y(ny)
    j=ny-1;
else
    j=1;
    while j<ny && yq>y(j+1)
        j=j+1;
    end
    if j>=ny
        j=ny-1;
    end
end
if zq<=z(1)
    k=1;
elseif zq>=z(nz)
    k=nz-1;
else
    k=1;
    while k<nz && zq>z(k+1)
        k=k+1;
    end
    if k>=nz
        k=nz-1;
    end
end
tx=0;
if x(i+1)>x(i)
    tx=(xq-x(i))/(x(i+1)-x(i));
end
ty=0;
if y(j+1)>y(j)
    ty=(yq-y(j))/(y(j+1)-y(j));
end
tz=0;
if z(k+1)>z(k)
    tz=(zq-z(k))/(z(k+1)-z(k));
end
c000=F(i,j,k);
c010=F(i,j+1,k);
c100=F(i+1,j,k);
c110=F(i+1,j+1,k);
c001=F(i,j,k+1);
c011=F(i,j+1,k+1);
c101=F(i+1,j,k+1);
c111=F(i+1,j+1,k+1);
c00=(1-tx)*c000+tx*c100;
c01=(1-tx)*c001+tx*c101;
c10=(1-tx)*c010+tx*c110;
c11=(1-tx)*c011+tx*c111;
c0=(1-ty)*c00+ty*c10;
c1=(1-ty)*c01+ty*c11;
v=(1-tz)*c0+tz*c1;
end
